simulink model "IARC_Nonlinear_Sensors"  (R2018a)
settings: Solver=ode1  StartTime=0.0  StopTime=20  FixedStep=T  RelTol=1e-3  EnableMultiTasking=on
undefined symbols (not defined in the file): A_1df, A_2df, alpha3, alpha_rp, alpha_x, alpha_z, an1, an1_v, an2, an3, bn1, bn1_v, bn2, bn3, dc_M_x, delta3, Epsilon3, F, g, Gamma1, Gamma2, Gamma3, Gamma4, gamma4_0, gamma_d_x, gamma_rp_0, gamma_x_0, gamma_z_0, Gammax, I, I_add, I_add_time, Jx, Jy, Jyaw, K, k1, k10, k11, k12, k2, k3, k4, k5, k6, k7, k8, k9, Ky, L, Light, LIMIT_CMD_PITCH, LIMIT_CMD_ROLL, LIMIT_CMD_xy, LIMIT_uCMD_HEIGHT, m, m_add, m_add_time, magnitude, MIL ... (+67)
libraries: simulink x131, simulink_extras x5, UAV_Control x4, aerolibwind2 x1
(part 1 of 6)
settings Model: Creator=ahmad  LastModifiedBy=Ahmad
settings SolverCC: AutoInsertRateTranBlk=on
settings DataIOCC: LimitDataPoints=on  SaveFormat=Array
settings OptimizationCC: LifeSpan=inf
settings DebuggingCC: UnderspecifiedInitializationDetection=Classic  MergeDetectMultiDrivingBlocksExec=none  SolverPrmCheckMsg=warning  StateNameClashWarn=warning  SFUnexpectedBacktrackingDiag=warning  SFNoUnconditionalDefaultTransitionDiag=warning  SFExecutionAtInitializationDiag=none
settings HardwareCC: ProdBitPerPointer=32  ProdBitPerSizeT=32  ProdBitPerPtrDiffT=32  ProdLargestAtomicFloat=None  ProdIntDivRoundTo=Undefined  ProdEndianess=Unspecified  ProdWordSize=32  ProdHWDeviceType=32-bit Generic
settings ModelReferenceCC: PropagateSignalLabelsOutOfModel=off
settings CodeAppCC: StateflowObjectComments=on
settings GRTTargetCC: TargetLangStandard=C89/C90 (ANSI)  GeneratePreprocessorConditionals=Disable all
settings ConfigComp: CovMetricSettings=dw  CovHtmlReporting=on  CovSaveCumulativeToWorkspaceVar=on  CovSaveSingleToWorkspaceVar=on  CovExternalEMLEnable=off

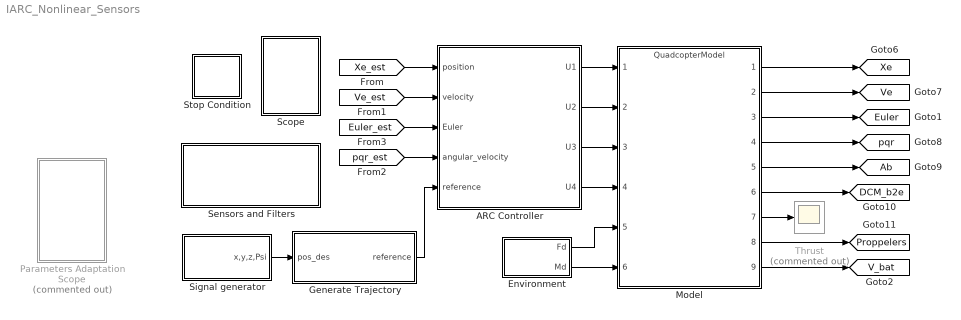
== system IARC_Nonlinear_Sensors ==
  ARC Controller : Subsystem
  Environment : Subsystem
  Generate Trajectory : Subsystem
  Model : ModelReference  ModelNameDialog=QuadcopterModel.slx  SimulationMode=Normal  ModelReferenceVersion=1.100
  Parameters Adaptation Scope : Subsystem  Commented=on
  Scope : Subsystem
  Sensors and Filters : Subsystem
  Signal generator : Subsystem
  Stop Condition : Subsystem
  Thrust : Scope  Commented=on
  tag scope: Ab=global, DCM_b2e=global, Euler=global, Proppelers=global, V_bat=global, Ve=global, Xe=global, pqr=global
  wires:
  Model/3 -> [Euler]
  ARC Controller/1(U1) -> Model/1
  ARC Controller/2(U2) -> Model/2
  ARC Controller/3(U3) -> Model/3
  ARC Controller/4(U4) -> Model/4
  Model/7 -> Thrust/1
  Generate Trajectory/1("reference ") -> ARC Controller/5("reference ")
  Model/4 -> [pqr]
  Model/6 -> [DCM_b2e]
  [Xe_est] -> ARC Controller/1(position)
  [Ve_est] -> ARC Controller/2(velocity)
  [Euler_est] -> ARC Controller/3(Euler)
  [pqr_est] -> ARC Controller/4(angular_velocity)
  Model/1 -> [Xe]
  Model/2 -> [Ve]
  Model/5 -> [Ab]
  Model/8 -> [Proppelers]
  Signal generator/1(x,y,z,Psi) -> Generate Trajectory/1(pos_des)
  Model/9 -> [V_bat]
  Environment/1(Fd) -> Model/5
  Environment/2(Md) -> Model/6

== system IARC_Nonlinear_Sensors/ARC Controller ==
  position : Inport
  velocity : Inport  Port=2
  Euler : Inport  Port=3
  angular_velocity : Inport  Port=4
  "reference " : Inport  Port=5
  Assign : Subsystem
  Attitutde Control : Subsystem
  Forces to decoupled PWM signals : Subsystem  AncestorBlock=UAV_Control/Forces to decoupled PWM signals  mask(Forces2PWMSignals){K=K, Ky=Ky, L=L}
      mask prompts: K "Proppeler Force Coefficient:"; Ky "Proppeler Torque Coefficient:"; L "Arm Length:"
      mask help: Convertes the Quadcopter desired forces and moments to equivalent PWM signal.
      mask Help:
      | Convertes the Quadcopter desired forces and moments to equivalent PWM signal for a specific motors configuration.
      | 
      | Motors indices and rotation direction:
      | 1: back (CW)
      | 2: front (CW)
      | 3: left (CCW)
      | 4: righ (CCW)
      | 
      | parameters:
      | K: Proppeler Force Coefficient (N/(rad/s)^2)
      | Ky: Proppeler Torque Coefficient (N.m/(rad/s)^2)
      | L: Arm Length (m)
      | 
      | Inputs:
      | Fn=F/(4K)
      | Txn=Tx/(2LK)
      | Tyn=Ty/(2LK)
      | Tzn=Tz/(4Ky)
      | 
      | Outputs:
      | u1 =sqrt( Fn + Tyn + Tzn)
      | u2 = sqrt(Fn - Tyn + Tzn)
      | u3 = sqrt(Fn + Txn - Tzn)
      | u4 = sqrt(Fn - Txn - Tzn)
      | 
      | The PWM Duty cylce (ui) is limeted between 0 and 1.
      mask Display:
      | port_label('input',1,'F_{z,des}','texmode','on')
      | port_label('input',2,'\tau_{x,des}','texmode','on')
      | port_label('input',3,'\tau_{y,des}','texmode','on')
      | port_label('input',4,'\tau_{z,des}','texmode','on')
      | port_label('output',1,'U_1','texmode','on')
      | port_label('output',2,'U_2','texmode','on')
      | port_label('output',3,'U_3','texmode','on')
      | port_label('output',4,'U_4','texmode','on')
  Gain1 : Gain
  Gain2 : Gain
  Gain3 : Gain
  LoT : Subsystem
  Mux : Mux
  Position Control : Subsystem
  Saturation1 : Saturate  UpperLimit=LIMIT_CMD_ROLL  LowerLimit=-LIMIT_CMD_ROLL
  Saturation2 : Saturate  UpperLimit=LIMIT_CMD_PITCH  LowerLimit=-LIMIT_CMD_PITCH
  "Thrust Initialization " : Subsystem  AncestorBlock=UAV_Control/Motors Initialization  mask(MotorsInitialization){t0=t0, t1=t1, Sat=Sat, Parameter4=Rate}
      mask prompts: t0 "Initialization delay:"; t1 "Input pass time:"; Sat "Signal saturation during initialization:"; Parameter4 "Signal rate during initialization:"
      mask help: Delays the pass out of the input while passing a warmup rizing signal.
      mask Display:
      | port_label('input',1,'u','texmode','on')
      | port_label('output',1,'y','texmode','on')
  To File4 : ToFile  Commented=on  Filename=U.mat  MatrixName=U  SaveFormat=Timeseries
  To Workspace : ToWorkspace  Commented=on  VariableName=U  SaveFormat=Timeseries  SampleTime=-1
  "U  " : Scope
  take-off flag : Subsystem
  "u1 " : Scope
  U1 : Outport
  U2 : Outport  Port=2
  U3 : Outport  Port=3
  U4 : Outport  Port=4
  tag scope: Fz_des=global, phi_d=global, theta_d=global
  wires:
  Forces to decoupled PWM signals/1(u1) -> Mux/1, U1/1
  Forces to decoupled PWM signals/2(u2) -> Mux/2, U2/1
  Forces to decoupled PWM signals/3(u3) -> Mux/3, U3/1
  Forces to decoupled PWM signals/4(u4) -> Mux/4, U4/1
  take-off flag/2(y2) -> Gain1/1
  Gain2/1 -> Forces to decoupled PWM signals/4(Tz_des)
  "Thrust Initialization "/1(y) -> LoT/1(u)
  take-off flag/3(y3) -> Gain2/1
  [z] -> take-off flag/4(h)
  Mux/1 -> To File4/1, To Workspace/1, "U  "/1
  take-off flag/1("y1 ") -> Gain3/1
  Position Control/2(phi_d) -> Saturation2/1
  Position Control/3(theta_d) -> Saturation1/1
  Saturation2/1 -> [phi_d], Attitutde Control/1(phi_d)
  Saturation1/1 -> [theta_d], Attitutde Control/2(theta_d)
  Attitutde Control/1(Tx) -> take-off flag/1("u1 ")
  Attitutde Control/2(Ty) -> take-off flag/2("u2 ")
  Attitutde Control/3(Tz) -> take-off flag/3(u3)
  Position Control/1(u_1) -> "Thrust Initialization "/1(u)
  LoT/1(y) -> "u1 "/1, [Fz_des], Forces to decoupled PWM signals/1(Fz_des)
  [psi_des] -> Attitutde Control/3(psi_d)
  Gain1/1 -> Forces to decoupled PWM signals/3(Ty_des)
  Gain3/1 -> Forces to decoupled PWM signals/2(Tx_des)
  position/1 -> Assign/1(position)
  velocity/1 -> Assign/2(velocity)
  Euler/1 -> Assign/3(Euler)
  angular_velocity/1 -> Assign/4(angular_velocity)
  "reference "/1 -> Assign/5("reference ")

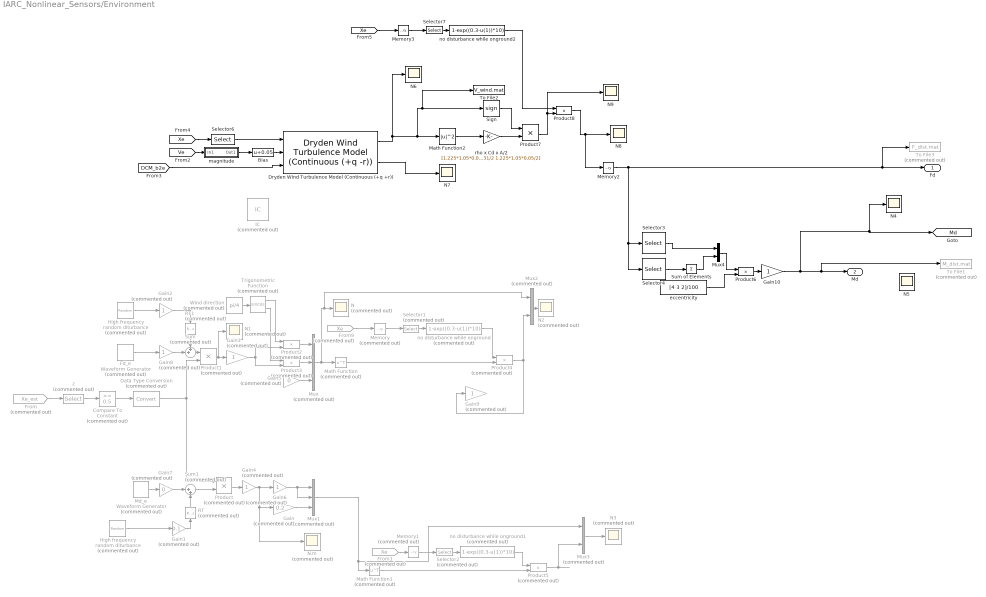
== system IARC_Nonlinear_Sensors/Environment ==
  Bias : Bias  Bias=0.05
  Compare To Constant : simulink/Logic and Bit Operations/Compare To Constant  Commented=on  relop=>=  const=0.5  OutDataTypeStr=boolean
  Data Type Conversion : DataTypeConversion  Commented=on
  Dryden Wind Turbulence Model (Continuous (+q +r)) : aerolibwind2/Dryden Wind Turbulence Model  (Continuous (+q -r))  units=Metric (MKS)  spec=MIL-F-8785C  model=Continuous Dryden (+q +r)  W20=25  Wdeg=30  TurbProb=10^-2 - Light  L_high=533.4  Wingspan=1.5  ts=0.1  Seed=[23341 23342 23443 13344]  T_on=on
      settings: SourceProductName=Aerospace Blockset
  Fd_e : simulink/Sources/Waveform Generator  Commented=on  OutMin=[]  OutMax=[]  OutDataTypeStr=double  SelectedSignal=1  Signals=-sin(0.5,pi/15,pi/3)  BlockNames=MultiportSwitch_6c45d7af92bb48a  SampleTime=T
      settings: SourceProductName=Simulink
  From : From  Commented=on  GotoTag=Xe_est  TagVisibility=global
  From1 : From  Commented=on  GotoTag=Xe  TagVisibility=global
  From9 : From  Commented=on  GotoTag=Xe  TagVisibility=global
  Gain : Gain  Commented=on  Gain=0.2
  Gain1 : Gain  Commented=on  Gain=0.1
  Gain10 : Gain
  Gain{2..4,6,8..9} (6 alike) : Gain  Commented=on
  Gain5 : Gain  Commented=on  Gain=0
  Gain7 : Gain  Commented=on  Gain=0
  High frequency random diturbance : RandomNumber  Commented=on  Variance=0.005  SampleTime=150*T
  "High frequency random diturbance " : RandomNumber  Commented=on  Variance=0.002  SampleTime=150*T
  IC : InitialCondition  Commented=on  Value=[1 0 0; 0 1 0; 0 0 1]
  Math Function : Math  Commented=on  Operator=transpose  SaturateOnIntegerOverflow=on
  Math Function1 : Math  Commented=on  Operator=transpose  SaturateOnIntegerOverflow=on
  Math Function2 : Math  Operator=magnitude^2  SaturateOnIntegerOverflow=on
  Md_e : simulink/Sources/Waveform Generator  Commented=on  OutMin=[]  OutMax=[]  OutDataTypeStr=double  SelectedSignal=1  Signals=sin(0.05,pi/10,0)+sin(0.0005,pi/4,0)#sin(0.001,10*pi,0)  BlockNames=MultiportSwitch_4e1e2af6a5c04c9#MultiportSwitch_b57f3ec1cbf3493  SampleTime=T
      settings: SourceProductName=Simulink
  Memory : Memory  Commented=on
  Memory1 : Memory  Commented=on
  Memory2 : Memory
  Memory3 : Memory
  Mux : Mux  Commented=on  Inputs=3
  Mux1 : Mux  Commented=on  Inputs=3
  Mux2 : Mux  Commented=on  Inputs=2
  Mux3 : Mux  Commented=on  Inputs=2
  Mux4 : Mux  Inputs=2
  N{,1..3} (4 alike) : Scope  Commented=on
  N.m : Scope  Commented=on
  N{4..9} (6 alike) : Scope
  Product{,1..5} (6 alike) : Product  Commented=on
  Product6 : Product
  Product7 : Product
  Product8 : Product
  RT : RateTransition  Commented=on  OutPortSampleTime=0.002
  RT1 : RateTransition  Commented=on  OutPortSampleTime=0.002
  Selector1 : Selector  Commented=on  InputPortWidth=3  IndexOptions=Index vector (dialog)  Indices=3  OutputSizes=1
  Selector2 : Selector  Commented=on  InputPortWidth=3  IndexOptions=Index vector (dialog)  Indices=3  OutputSizes=1
  Selector3 : Selector  InputPortWidth=3  IndexOptions=Index vector (dialog)  Indices=[2 1]  OutputSizes=1
  Selector4 : Selector  InputPortWidth=3  IndexOptions=Index vector (dialog)  Indices=[2 1]  OutputSizes=1
  Selector6 : Selector  InputPortWidth=3  IndexOptions=Index vector (dialog)  Indices=3  OutputSizes=1
  Selector7 : Selector  InputPortWidth=3  IndexOptions=Index vector (dialog)  Indices=3  OutputSizes=1
  Sign : Signum
  Sum : Sum  Commented=on  Inputs=++|
  Sum of Elements : Sum  Inputs=+
  Sum1 : Sum  Commented=on  Inputs=|++
  To File1 : ToFile  Commented=on  Filename=M_dist.mat  MatrixName=M_dist  SaveFormat=Timeseries
  To File2 : ToFile  Filename=V_wind.mat  MatrixName=V_wind  SaveFormat=Timeseries
  To File3 : ToFile  Commented=on  Filename=F_dist.mat  MatrixName=F_dist  SaveFormat=Timeseries
  Trigonometric Function : Trigonometry  Commented=on  Operator=sincos
  Wind direction : Constant  Commented=on  Value=pi/4
  eccentricity : Constant  Value=[4 3 2]/100
  magnitude : Subsystem
  no disturbance while onground : Fcn  Commented=on  Expr=1-exp((0.3-u(1))*10)
  no disturbance while onground1 : Fcn  Commented=on  Expr=1-exp((0.3-u(1))*10)
  no disturbance while onground2 : Fcn  Expr=1-exp((0.3-u(1))*10)
  rho x Cd x A/2 : Gain  Gain=[1.225*1.05*0.0331/2 1.225*1.05*0.0331/2 1.225*1.05*0.05/2]
  z : Selector  Commented=on  InputPortWidth=3  IndexOptions=Index vector (dialog)  Indices=3  OutputSizes=1
  Fd : Outport
  Md : Outport  Port=2
  tag scope: Md=global
  wires:
  From/1 -> z/1
  Compare To Constant/1 -> Data Type Conversion/1
  z/1 -> Compare To Constant/1
  Sum1/1 -> Product/2
  Data Type Conversion/1 -> Product1/2, Product/1
  Fd_e/1 -> Gain8/1
  Mux/1 -> Mux2/1, N/1, Math Function/1
  Mux1/1 -> Math Function1/1, Mux3/1
  Product4/1 -> Mux2/2, Gain9/1
  Product/1 -> Gain4/1
  High frequency random diturbance/1 -> Gain2/1
  Sum/1 -> Product1/1
  Md_e/1 -> Gain7/1
  "High frequency random diturbance "/1 -> Gain1/1
  RT/1 -> Sum1/2
  RT1/1 -> Sum/1
  Gain/1 -> Mux1/3
  Gain1/1 -> RT/1
  Gain2/1 -> RT1/1
  Gain4/1 -> Gain6/1, Gain/1, N.m/1
  Gain5/1 -> Mux/3
  Wind direction/1 -> Trigonometric Function/1
  Product2/1 -> Mux/1
  Product3/1 -> Mux/2
  Trigonometric Function/1 -> Product2/1
  Trigonometric Function/2 -> Product3/1
  Gain3/1 -> Product3/2, Product2/2
  Product1/1 -> N1/1, Gain3/1
  Gain6/1 -> Mux1/2, Mux1/1
  Math Function/1 -> Product4/2
  From9/1 -> Memory/1
  Selector1/1 -> no disturbance while onground/1
  no disturbance while onground/1 -> Product4/1
  no disturbance while onground1/1 -> Product5/1
  Selector2/1 -> no disturbance while onground1/1
  From1/1 -> Memory1/1
  Math Function1/1 -> Product5/2
  Memory/1 -> Selector1/1
  Memory1/1 -> Selector2/1
  Product5/1 -> Mux3/2
  Mux2/1 -> N2/1
  Mux3/1 -> N3/1
  Gain7/1 -> Sum1/1
  Gain8/1 -> Sum/2
  Product6/1 -> Gain10/1
  eccentricity/1 -> Product6/2
  Selector3/1 -> Mux4/1
  Selector4/1 -> Sum of Elements/1
  Mux4/1 -> Product6/1
  Sum of Elements/1 -> Mux4/2
  Gain10/1 -> N4/1, [Md], To File1/1, Md/1
  magnitude/1(Out1) -> Bias/1
  Dryden Wind Turbulence Model (Continuous (+q +r))/2 -> N7/1
  [Xe] -> Selector6/1
  [Ve] -> magnitude/1(In1)
  Selector6/1 -> Dryden Wind Turbulence Model (Continuous (+q +r))/1
  Dryden Wind Turbulence Model (Continuous (+q +r))/1 -> N6/1, To File2/1, Sign/1, Math Function2/1
  [DCM_b2e] -> Dryden Wind Turbulence Model (Continuous (+q +r))/3
  Bias/1 -> Dryden Wind Turbulence Model (Continuous (+q +r))/2
  Math Function2/1 -> rho x Cd x A/2/1
  rho x Cd x A/2/1 -> Product7/2
  Sign/1 -> Product7/1
  Memory3/1 -> Selector7/1
  no disturbance while onground2/1 -> Product8/1
  Selector7/1 -> no disturbance while onground2/1
  [Xe] -> Memory3/1
  Product8/1 -> N8/1, Memory2/1
  Product7/1 -> N9/1, Product8/2
  Memory2/1 -> To File3/1, Fd/1, Selector4/1, Selector3/1

== system IARC_Nonlinear_Sensors/Generate Trajectory ==
  pos_des : Inport
  Bias : Bias  Commented=on  Bias=-15
  Bias1 : Bias  Bias=Zg
  Clock2 : Clock  Commented=on
  Compare To Constant1 : simulink/Logic and Bit Operations/Compare To Constant  Commented=on  relop=>=  const=15  OutDataTypeStr=boolean
  Compare To Constant2 : simulink/Logic and Bit Operations/Compare To Constant  Commented=on  relop=<=  const=20  OutDataTypeStr=boolean
  Demux : Demux
  Logical Operator : Logic  Commented=on  AllPortsSameDT=off  OutDataTypeStr=boolean
  Mux : Mux
  Product1 : Product  Commented=on
  Rate Limiter1 : RateLimiter
  Rate Limiter2 : RateLimiter
  Rate Limiter3 : RateLimiter  RisingSlewLimit=2  FallingSlewLimit=-2
  Sine Wave2 : Sin  Commented=on  TimeSource=Use external signal  Frequency=2*pi  SampleTime=0
  Sum4 : Sum  Inputs=++|
  Transfer Fcn11 : TransferFcn  Denominator=conv(conv(conv([0.2 1],[0.2 1]),[0.2 1]),[0.2 1])
  Transfer Fcn14 : TransferFcn  Denominator=conv(conv(conv([0.2 1],[0.2 1]),[0.2 1]),[0.2 1])
  Transfer Fcn17 : TransferFcn  Denominator=conv([0.2 1],[0.2 1])
  Transfer Fcn6 : TransferFcn  Denominator=conv(conv(conv([0.2 1],[0.2 1]),[0.2 1]),[0.2 1])
  Transfer Fcn8 : TransferFcn  Commented=on  Denominator=conv(conv(conv(conv(conv(conv(conv([0.2 1],[0.2 1]),[0.2 1]),[0.2 1]),[0.2 1]),[0.2 1]),[0.2 1]),[0.2 1])
  adjust_for_heading3 : Subsystem  Commented=on
  des psi : Scope  Commented=on
  des x : Scope  Commented=on
  des x3 : Scope  Commented=on
  des y : Scope  Commented=on
  des z : Scope  Commented=on
  steady takeoff (x) : Subsystem  Commented=on
  steady takeoff (y) : Subsystem  Commented=on
  "reference " : Outport
  wires:
  Bias1/1 -> des z/1, Mux/3  "z_des"
  Demux/2 -> Rate Limiter1/1  "y_des"
  pos_des/1 -> Demux/1
  Sum4/1 -> Mux/1, des x/1
  Product1/1 -> Transfer Fcn8/1
  Clock2/1 -> Compare To Constant2/1, Bias/1, Compare To Constant1/1
  Logical Operator/1 -> Product1/2
  Sine Wave2/1 -> Product1/1
  Transfer Fcn8/1 -> ?
  Bias/1 -> Sine Wave2/1
  Compare To Constant2/1 -> Logical Operator/1
  Compare To Constant1/1 -> Logical Operator/2
  Demux/4 -> Transfer Fcn17/1  "psi_des"
  Demux/1 -> Rate Limiter2/1, des x3/1  "x_des"
  Mux/1 -> "reference "/1
  Demux/3 -> Rate Limiter3/1  "z_des"
  Transfer Fcn11/1 -> Bias1/1  "z_des"
  Rate Limiter3/1 -> Transfer Fcn11/1
  Rate Limiter2/1 -> Transfer Fcn6/1  "x_des"
  Transfer Fcn6/1 -> Sum4/2
  Transfer Fcn14/1 -> Mux/2, des y/1
  Rate Limiter1/1 -> Transfer Fcn14/1  "y_des"
  Transfer Fcn17/1 -> Mux/4, des psi/1

== system IARC_Nonlinear_Sensors/Parameters Adaptation Scope ==
  Mux{,1..4} (5 alike) : Mux
  Subsystem : Subsystem
  Subsystem1 : Subsystem
  Subsystem2 : Subsystem
  m : Scope
  max : Constant  Value=theta1_Max
  max1 : Constant  Value=theta2_Max
  max2 : Constant  Value=theta3_Max(1)
  max3 : Constant  Value=theta4_Max
  max4 : Constant  Value=theta3_Max(2)
  min : Constant  Value=theta1_Min
  min1 : Constant  Value=theta2_Min
  min2 : Constant  Value=theta3_Min(1)
  min3 : Constant  Value=theta4_Min
  min4 : Constant  Value=theta3_Min(2)
  real : Constant  Value=theta1
  real1 : Constant  Value=theta2
  real2 : Constant  Value=theta3(1)
  real3 : Constant  Value=theta4
  real4 : Constant  Value=theta3(2)
  theta1 1/Iy : Scope
  theta2 1/Ix : Scope
  theta3_1 1/m : Scope
  theta3_2 d0 : Scope
  theta4 1/Iz : Scope
  wires:
  min1/1 -> Mux1/4
  max1/1 -> Mux1/1
  real2/1 -> Mux2/2
  Mux1/1 -> theta2 1/Ix/1
  Mux2/1 -> Subsystem2/1(" "), Subsystem/1(" ")
  max2/1 -> Mux2/1
  min2/1 -> Mux2/4
  [theta2_est] -> Mux1/3
  real1/1 -> Mux1/2
  Mux/1 -> theta1 1/Iy/1
  real/1 -> Mux/2
  [theta4_est] -> Mux3/3
  [theta1_est] -> Mux/3
  min/1 -> Mux/4
  Mux3/1 -> theta4 1/Iz/1
  max3/1 -> Mux3/1
  real3/1 -> Mux3/2
  min3/1 -> Mux3/4
  max/1 -> Mux/1
  real4/1 -> Mux4/2
  Mux4/1 -> Subsystem1/1(" ")
  max4/1 -> Mux4/1
  min4/1 -> Mux4/4
  [theta3_est] -> Mux2/3
  [theta3_est] -> Mux4/3
  Subsystem/1("  ") -> m/1
  Subsystem1/1("  ") -> theta3_2 d0/1
  Subsystem2/1("  ") -> theta3_1 1/m/1

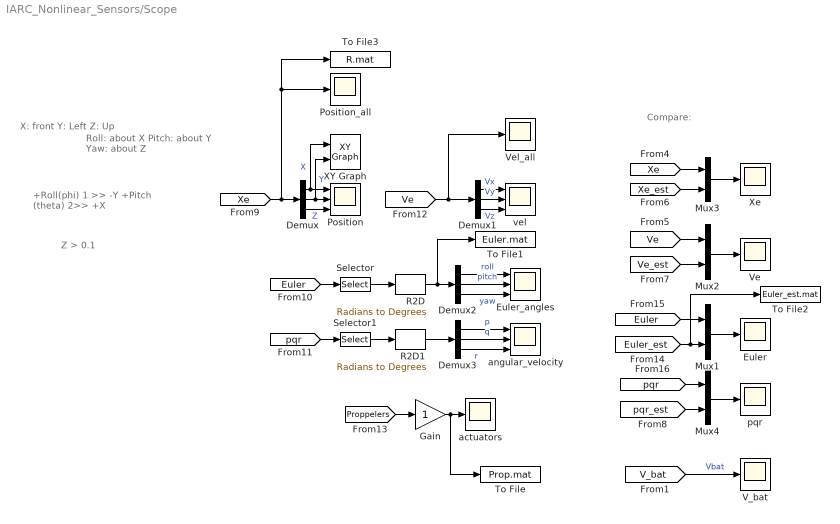
== system IARC_Nonlinear_Sensors/Scope ==
  note: Compare:
  note: +Roll(phi) 1 >> -Y
      | +Pitch (theta) 2>> +X
  note: Roll: about X
      | Pitch: about Y
      | Yaw: about Z
  note: Z > 0.1
  note: X: front
      | Y: Left
      | Z: Up
  Demux{,1..3} (4 alike) : Demux  Outputs=3
  "Euler " : Scope
  Euler_angles : Scope  NumInputPorts=3
  Gain : Gain
  Mux{1..4} (4 alike) : Mux  Inputs=2
  Position : Scope  NumInputPorts=3
  Position_all : Scope
  R2D : simulink_extras/Transformations/Radians to Degrees
  R2D1 : simulink_extras/Transformations/Radians to Degrees
  Selector : Selector  InputPortWidth=3  IndexOptions=Index vector (dialog)  Indices=[1 2 3]  OutputSizes=1
  Selector1 : Selector  InputPortWidth=3  IndexOptions=Index vector (dialog)  Indices=[1 2 3]  OutputSizes=1
  To File : ToFile  Filename=Prop.mat  MatrixName=Prop  SaveFormat=Timeseries
  To File1 : ToFile  Filename=Euler.mat  MatrixName=Euler  SaveFormat=Timeseries
  To File2 : ToFile  Filename=Euler_est.mat  MatrixName=Euler_est  SaveFormat=Timeseries
  To File3 : ToFile  Filename=R.mat  MatrixName=R  SaveFormat=Timeseries
  V_bat : Scope
  Ve : Scope
  Vel_all : Scope
  XY Graph : simulink/Sinks/XY Graph  xmin=-3  xmax=3  ymin=-3  ymax=3  st=1/100
  Xe : Scope
  actuators : Scope
  angular_velocity : Scope  NumInputPorts=3
  "pqr " : Scope
  vel : Scope  NumInputPorts=3
  wires:
  [pqr_est] -> Mux4/2
  Mux1/1 -> "Euler "/1
  [Euler] -> Selector/1
  [Ve] -> Vel_all/1, Demux1/1
  Demux2/3 -> Euler_angles/3  "yaw"
  [Xe_est] -> Mux3/2
  [Euler] -> Mux1/1
  [pqr] -> Selector1/1
  Mux4/1 -> "pqr "/1
  Selector1/1 -> R2D1/1
  [Ve] -> Mux2/1
  [Xe] -> To File3/1, Position_all/1, Demux/1
  [Proppelers] -> Gain/1
  Mux2/1 -> Ve/1
  Demux2/1 -> Euler_angles/1  "roll"
  Mux3/1 -> Xe/1
  Demux3/3 -> angular_velocity/3  "r"
  R2D1/1 -> Demux3/1
  Selector/1 -> R2D/1
  Demux1/1 -> vel/1  "Vx"
  Demux1/2 -> vel/2  "Vy"
  [Ve_est] -> Mux2/2
  Demux3/2 -> angular_velocity/2  "q"
  Gain/1 -> To File/1, actuators/1
  [pqr] -> Mux4/1
  Demux/3 -> Position/3  "Z"
  Demux/1 -> Position/1, XY Graph/1  "X"
  Demux1/3 -> vel/3  "Vz"
  R2D/1 -> To File1/1, Demux2/1
  [Xe] -> Mux3/1
  Demux3/1 -> angular_velocity/1  "p"
  Demux/2 -> XY Graph/2, Position/2  "Y"
  Demux2/2 -> Euler_angles/2  "pitch"
  [Euler_est] -> To File2/1, Mux1/2
  [V_bat] -> V_bat/1  "Vbat"

== system IARC_Nonlinear_Sensors/Sensors and Filters ==
  Data processing : Subsystem
  Rotation Angles to Angular transformation matrix earth to body Rotation Order: ZXY : UAV_Control/Rotation Angles to Angular transformation matrix earth to body Rotation Order: ZXY
      settings: SourceProductName=UAV_Control
  Sensors : Subsystem
  tag scope: Euler_est=global, Rr_est=global, Ve_est=global, Xe_est=global, pqr_est=global, pqr_gyro=global
  wires:
  Data processing/4("p,q,r_est ") -> [pqr_est]
  [Euler] -> Sensors/4(Euler)
  Sensors/3("p,q,r ") -> Data processing/3(p,q,r)
  [pqr] -> Sensors/1(p,q,r)
  [Xe] -> Sensors/3(Xe)
  [DCM_b2e] -> Sensors/5(DCM_b2e)
  Sensors/1(Acc) -> Data processing/1(Acc)
  Sensors/2(OptiTrack) -> Data processing/2(OptiTrack)
  Data processing/2(Ve_est) -> [Ve_est]
  Data processing/1(Xe_est) -> [Xe_est]
  [Ab] -> Sensors/2(Ab)
  Data processing/3(p,q,r_gyro) -> [pqr_gyro]
  Rotation Angles to Angular transformation matrix earth to body Rotation Order: ZXY/1 -> [Rr_est]
  Data processing/5(" Euler_est") -> Rotation Angles to Angular transformation matrix earth to body Rotation Order: ZXY/1, [Euler_est]

== system IARC_Nonlinear_Sensors/Signal generator ==
  Mux1 : Mux
  Position2 : Scope  Commented=on
  Rate Transition : RateTransition  Commented=on
  Repeating Sequence Stair : simulink/Sources/Repeating Sequence Stair  Commented=on  OutValues=[0 0 1 0 0 -1 0 1].'  tsamp=T*500*5  OutMin=[]  OutMax=[]  OutDataTypeStr=double  OutputDataTypeScalingMode=double  OutDataType=fixdt(0,8)  ConRadixGroup=Best Precision: Vector-wise  OutScaling=2^-12
  X Des : Scope  Commented=on
  X_des : Subsystem
  Y Des : Scope  Commented=on
  Y_des : Subsystem
  Yaw_des : Subsystem
  Z_des : Subsystem
  x,y,z,Psi : Outport
  wires:
  Rate Transition/1 -> Position2/1
  Repeating Sequence Stair/1 -> Rate Transition/1  "y_des"
  Mux1/1 -> x,y,z,Psi/1
  Z_des/1(z_des) -> Mux1/3
  X_des/1(x_des) -> X Des/1, Mux1/1
  Y_des/1(x_des) -> Y Des/1, Mux1/2
  Yaw_des/1(Out1) -> Mux1/4

== system IARC_Nonlinear_Sensors/Stop Condition ==
  Abs : Abs
  Abs1 : Abs
  Assertion : Assertion  AssertionFailFcn=msgbox('Low Voltage!')
  Assertion1 : Assertion  AssertionFailFcn=msgbox('Crash!')
  Compare To Constant : simulink/Logic and Bit Operations/Compare To Constant  relop=>=  const=3.0  OutDataTypeStr=boolean
  Compare To Constant1 : simulink/Logic and Bit Operations/Compare To Constant  relop=>=  const=3.0  OutDataTypeStr=boolean
  Compare To Constant2 : simulink/Logic and Bit Operations/Compare To Constant  relop=>=  const=3.0  OutDataTypeStr=boolean
  Compare To Constant3 : simulink/Logic and Bit Operations/Compare To Constant  relop=<=  const=Zg  OutDataTypeStr=boolean
  Compare To Constant4 : simulink/Logic and Bit Operations/Compare To Constant  relop=<  const=-1  OutDataTypeStr=boolean
  Compare To Constant5 : simulink/Logic and Bit Operations/Compare To Constant  relop=>=  const=Zg+10/100  OutDataTypeStr=boolean
  Compare To Constant6 : simulink/Logic and Bit Operations/Compare To Constant  relop=<  const=9  OutDataTypeStr=boolean
  Demux : Demux  Outputs=3
  Logical Operator : Logic  Inputs=3  AllPortsSameDT=off  OutDataTypeStr=boolean
  Logical Operator1 : Logic  Operator=OR  Inputs=4  AllPortsSameDT=off  OutDataTypeStr=boolean
  Logical Operator2 : Logic  Operator=NOT  AllPortsSameDT=off  OutDataTypeStr=boolean
  Logical Operator3 : Logic  Operator=NOT  AllPortsSameDT=off  OutDataTypeStr=boolean
  Vz : Selector  InputPortWidth=3  IndexOptions=Index vector (dialog)  Indices=3  OutputSizes=1
  st : Scope  Commented=on
  wires:
  Demux/1 -> Abs/1
  Compare To Constant/1 -> Logical Operator1/1
  Vz/1 -> Compare To Constant4/1
  Demux/3 -> Compare To Constant3/1, Compare To Constant2/1
  Compare To Constant3/1 -> Logical Operator/1
  Abs/1 -> Compare To Constant/1
  [Xe] -> Demux/1
  Compare To Constant1/1 -> Logical Operator1/2
  Abs1/1 -> Compare To Constant1/1
  Logical Operator1/1 -> Logical Operator2/1
  Demux/2 -> Abs1/1
  Logical Operator/1 -> st/1, Logical Operator1/4
  Compare To Constant2/1 -> Logical Operator1/3
  Compare To Constant4/1 -> Logical Operator/2
  [Ve] -> Vz/1
  [z_des] -> Compare To Constant5/1
  Compare To Constant5/1 -> Logical Operator/3
  [V_bat] -> Compare To Constant6/1
  Compare To Constant6/1 -> Logical Operator3/1
  Logical Operator2/1 -> Assertion1/1
  Logical Operator3/1 -> Assertion/1

== system IARC_Nonlinear_Sensors/ARC Controller/Assign ==
  position : Inport
  velocity : Inport  Port=2
  Euler : Inport  Port=3
  angular_velocity : Inport  Port=4
  "reference " : Inport  Port=5
  Demux{,1,3..4} (4 alike) : Demux  Outputs=3
  Demux2 : Demux
  tag scope: phi=global, phi_dot=global, psi=global, psi_des=global, psi_dot=global, theta=global, theta_dot=global, x=global, x_des=global, x_dot=global, y=global, y_des=global, y_dot=global, z=global, z_des=global, z_dot=global
  wires:
  position/1 -> Demux/1
  Demux2/1 -> [x_des]
  Demux1/3 -> [psi]
  Demux1/2 -> [theta]
  Demux/3 -> [z]
  Euler/1 -> Demux1/1
  Demux4/3 -> [z_dot]
  "reference "/1 -> Demux2/1
  Demux2/4 -> [psi_des]
  Demux3/3 -> [psi_dot]
  Demux/2 -> [y]
  velocity/1 -> Demux4/1
  Demux3/1 -> [phi_dot]
  Demux4/2 -> [y_dot]
  Demux1/1 -> [phi]
  Demux4/1 -> [x_dot]
  Demux/1 -> [x]
  Demux2/2 -> [y_des]
  Demux2/3 -> [z_des]
  Demux3/2 -> [theta_dot]
  angular_velocity/1 -> Demux3/1

== system IARC_Nonlinear_Sensors/ARC Controller/Attitutde Control ==
  phi_d : Inport
  theta_d : Inport  Port=2
  psi_d : Inport  Port=3
  Add : Sum  Commented=on  Inputs=--+-++
  Product : Product  Commented=on  Multiplication=Matrix(*)
  Product1 : Product  Commented=on  Multiplication=Matrix(*)
  Product2 : Product  Commented=on  Multiplication=Matrix(*)
  Subsystem : Subsystem  Commented=on
  Yaw control : Subsystem
  pitch control : Subsystem
  roll control : Subsystem
  u_{1..8} (8 alike) : Scope  Commented=on
  Tx : Outport
  Ty : Outport  Port=2
  Tz : Outport  Port=3
  wires:
  theta_d/1 -> pitch control/1(theta_d)
  phi_d/1 -> roll control/1(phi_d)
  Subsystem/1("inv(g) ") -> u_4/1, Product/1
  Subsystem/2("f ") -> u_1/1, Add/1
  Subsystem/3(D) -> u_6/1, Add/2
  Product1/1 -> u_5/1, Add/3
  Subsystem/4(k1) -> Product1/1
  Subsystem/6(e1) -> Product1/2, u_8/1, Add/5
  Product2/1 -> u_7/1, Add/4
  Subsystem/5(k2) -> Product2/1
  Subsystem/7(e2) -> Product2/2
  Add/1 -> Product/2
  Subsystem/8(X_ddot) -> u_3/1, Add/6
  Product/1 -> u_2/1
  roll control/1(U4 (N.m)) -> Tx/1
  pitch control/1(U5 (N.m)) -> Ty/1
  psi_d/1 -> Yaw control/1(psi_d)
  Yaw control/1(U6 (N.m)) -> Tz/1

== system IARC_Nonlinear_Sensors/ARC Controller/Forces to decoupled PWM signals ==
  Fz_des : Inport
  Tx_des : Inport  Port=2
  Ty_des : Inport  Port=3
  Tz_des : Inport  Port=4
  Gain : Gain  Commented=on  Gain=1/2
  Gain1 : Gain  Commented=on  Gain=1/4
  Gain2 : Gain  Gain=1/(L*2*K)
  Gain3 : Gain  Gain=1/(4*Ky)
  Gain4 : Gain  Gain=1/(L*2*K)
  Gain5 : Gain  Gain=1/(4*K)
  Gain6 : Gain  Commented=on  Gain=1/2
  Gain7 : Gain  Commented=on  Gain=1/4
  Mux : Mux
  Saturation{1..4} (4 alike) : Saturate  UpperLimit=1  LowerLimit=0
  Sqrt{,1..3} (4 alike) : Sqrt  Operator=signedSqrt  OutputSignalType=real  SaturateOnIntegerOverflow=on
  u1^2 - Back (PWM command) : Fcn  Expr=u(1)+u(3)+u(4)
  u2^2 - Front (PWM command) : Fcn  Expr=u(1)-u(3)+u(4)
  u3^2 - Left (PWM command) : Fcn  Expr=u(1)+u(2)-u(4)
  u4^2 - Right (PWM command) : Fcn  Expr=u(1)-u(2)-u(4)
  u1 : Outport
  u2 : Outport  Port=2
  u3 : Outport  Port=3
  u4 : Outport  Port=4
  wires:
  Tx_des/1 -> Gain2/1
  Fz_des/1 -> Gain5/1
  Ty_des/1 -> Gain4/1
  Tz_des/1 -> Gain3/1
  Mux/1 -> u4^2 - Right (PWM command)/1, u3^2 - Left (PWM command)/1, u2^2 - Front (PWM command)/1, u1^2 - Back (PWM command)/1
  Gain2/1 -> Mux/2
  Gain4/1 -> Mux/3
  Gain3/1 -> Mux/4
  Gain5/1 -> Mux/1
  Saturation4/1 -> u1/1
  Saturation2/1 -> u3/1
  Saturation3/1 -> u2/1
  Saturation1/1 -> u4/1
  u1^2 - Back (PWM command)/1 -> Sqrt/1
  u2^2 - Front (PWM command)/1 -> Sqrt1/1
  u3^2 - Left (PWM command)/1 -> Sqrt2/1
  u4^2 - Right (PWM command)/1 -> Sqrt3/1
  Sqrt/1 -> Saturation4/1
  Sqrt3/1 -> Saturation1/1
  Sqrt2/1 -> Saturation2/1
  Sqrt1/1 -> Saturation3/1

== system IARC_Nonlinear_Sensors/ARC Controller/LoT ==
  u : Inport
  Gain : Gain  Gain=0
  Product : Product
  Step : Step  Time=40  SampleTime=0
  Sum : Sum  Inputs=-+|
  y : Outport
  wires:
  Step/1 -> Product/1
  Product/1 -> Sum/1
  u/1 -> Gain/1, Sum/2
  Sum/1 -> y/1
  Gain/1 -> Product/2

== system IARC_Nonlinear_Sensors/ARC Controller/Position Control ==
  Coupling : Subsystem
  X control : Subsystem
  Y control : Subsystem
  Z control : Subsystem
  phi_des : Scope
  theta_des : Scope
  u1 : Scope
  u_1 : Outport
  phi_d : Outport  Port=2
  theta_d : Outport  Port=3
  wires:
  [psi_des] -> Coupling/4(psi_d)
  X control/1(U1 (m/s^2)) -> Coupling/1(U1)
  Y control/1(U2 (m/s^2)) -> Coupling/2(U2)
  Z control/1(U3 (m/s^2)) -> Coupling/3(U3)
  Coupling/2(phi_d (rad)) -> phi_d/1, phi_des/1
  Coupling/3(theta_d (rad)) -> theta_des/1, theta_d/1
  Coupling/1(u1 (N)) -> u_1/1, u1/1

== system IARC_Nonlinear_Sensors/ARC Controller/Thrust Initialization  ==
  u : Inport
  Clock : Clock
  Compare To Constant1 : simulink/Logic and Bit Operations/Compare To Constant  relop=<=  const=t1  OutDataTypeStr=boolean
  Compare To Constant2 : simulink/Logic and Bit Operations/Compare To Constant  relop=>=  const=t0  OutDataTypeStr=boolean
  Constant : Constant  Value=0
  Gain : Gain  Gain=Rate
  Saturation : Saturate  UpperLimit=Sat  LowerLimit=0
  Scope : Scope
  Scope1 : Scope
  Switch : Switch  Criteria=u2 > Threshold  Threshold=0.5
  Switch1 : Switch  Criteria=u2 > Threshold  Threshold=0.5
  y : Outport
  wires:
  Switch/1 -> Scope/1, Switch1/1
  Switch1/1 -> y/1, Scope1/1
  Compare To Constant1/1 -> Switch1/2
  Constant/1 -> Switch/3
  Saturation/1 -> Switch/1
  Gain/1 -> Saturation/1
  Compare To Constant2/1 -> Switch/2
  Clock/1 -> Gain/1, Compare To Constant2/1, Compare To Constant1/1
  u/1 -> Switch1/3

== system IARC_Nonlinear_Sensors/ARC Controller/take-off flag ==
  "u1 " : Inport
  "u2 " : Inport  Port=2
  u3 : Inport  Port=3
  h : Inport  Port=4
  Constant : Constant  Value=[0 0 0]
  Demux : Demux  Outputs=3
  Mux : Mux  Inputs=3
  Switch : Switch  Criteria=u2 > Threshold  Threshold=X0(3)+2/100
  "y1 " : Outport
  y2 : Outport  Port=2
  y3 : Outport  Port=3
  wires:
  Constant/1 -> Switch/3
  Demux/1 -> "y1 "/1
  Mux/1 -> Switch/1
  "u1 "/1 -> Mux/1
  "u2 "/1 -> Mux/2
  u3/1 -> Mux/3
  h/1 -> Switch/2
  Switch/1 -> Demux/1
  Demux/3 -> y3/1
  Demux/2 -> y2/1

== system IARC_Nonlinear_Sensors/Environment/magnitude ==
  In1 : Inport
  Math Function2 : Math  Operator=magnitude^2  SaturateOnIntegerOverflow=on
  Sqrt : Sqrt  SaturateOnIntegerOverflow=on
  Sum of Elements1 : Sum  Inputs=+
  Out1 : Outport
  wires:
  Sum of Elements1/1 -> Sqrt/1
  Math Function2/1 -> Sum of Elements1/1
  Sqrt/1 -> Out1/1
  In1/1 -> Math Function2/1

== system IARC_Nonlinear_Sensors/Generate Trajectory/adjust_for_heading3 ==
  x_w_des : Inport
  y_w_des : Inport  Port=2
  adjust_for_heading1 : Subsystem
  adjust_for_heading3 : Subsystem
  x_des_adj : Outport
  y_des_adj : Outport  Port=2
  wires:
  y_w_des/1 -> adjust_for_heading3/2(y_e_d), adjust_for_heading1/2(y_e_d)
  [psi] -> adjust_for_heading3/3(yaw), adjust_for_heading1/3(yaw)
  x_w_des/1 -> adjust_for_heading3/1(x_e_d), adjust_for_heading1/1(x_e_d)
  adjust_for_heading1/1(adj) -> x_des_adj/1
  adjust_for_heading3/1(adj) -> y_des_adj/1

== system IARC_Nonlinear_Sensors/Generate Trajectory/steady takeoff (x) ==
  u : Inport
  Compare To Constant : simulink/Logic and Bit Operations/Compare To Constant  relop=>=  const=Safe_hight  OutDataTypeStr=boolean
  Data Type Conversion : DataTypeConversion
  Mux : Mux  Inputs=3
  Switch : Switch  Criteria=u2 > Threshold  Threshold=0.5
  Triggered Subsystem1 : Subsystem  TreatAsAtomicUnit=on
  Triggered Subsystem2 : Subsystem  TreatAsAtomicUnit=on
  start from initial position : Sum  Inputs=|++
  z_des{1,4..5,7} (4 alike) : Scope
  y : Outport
  wires:
  Triggered Subsystem2/1("  ") -> z_des7/1, Mux/2, Switch/3, start from initial position/2
  [takeoff] -> Triggered Subsystem2/Trigger
  start from initial position/1 -> Mux/1, Switch/1
  [z] -> Compare To Constant/1
  Switch/1 -> Mux/3, y/1
  [x] -> Triggered Subsystem2/1(" "), z_des5/1
  Triggered Subsystem1/1("  ") -> z_des4/1, Switch/2
  Compare To Constant/1 -> Data Type Conversion/1
  Data Type Conversion/1 -> Triggered Subsystem1/Trigger, Triggered Subsystem1/1(" ")
  Mux/1 -> z_des1/1
  u/1 -> start from initial position/1

== system IARC_Nonlinear_Sensors/Generate Trajectory/steady takeoff (y) ==
  u : Inport
  Compare To Constant : simulink/Logic and Bit Operations/Compare To Constant  relop=>=  const=Safe_hight  OutDataTypeStr=uint8
  Data Type Conversion : DataTypeConversion
  Switch : Switch  Criteria=u2 > Threshold  Threshold=0.5
  Triggered Subsystem1 : Subsystem  TreatAsAtomicUnit=on
  Triggered Subsystem2 : Subsystem  TreatAsAtomicUnit=on
  start from initial position : Sum  Inputs=|++
  z_des4 : Scope
  z_des5 : Scope
  z_des7 : Scope
  y : Outport
  wires:
  Compare To Constant/1 -> Data Type Conversion/1
  Triggered Subsystem1/1("  ") -> Switch/2, z_des4/1
  [y] -> Triggered Subsystem2/1(" "), z_des5/1
  Switch/1 -> y/1
  [z] -> Compare To Constant/1
  start from initial position/1 -> Switch/1
  [takeoff] -> Triggered Subsystem2/Trigger
  Triggered Subsystem2/1("  ") -> start from initial position/2, Switch/3, z_des7/1
  Data Type Conversion/1 -> Triggered Subsystem1/Trigger, Triggered Subsystem1/1(" ")
  u/1 -> start from initial position/1

== system IARC_Nonlinear_Sensors/Parameters Adaptation Scope/Subsystem ==
  " " : Inport
  Demux : Demux  Outputs=5
  Math Function1 : Math  Operator=reciprocal  SaturateOnIntegerOverflow=on
  Mux5 : Mux
  Terminator : Terminator
  "  " : Outport
  wires:
  Demux/2 -> Mux5/2
  " "/1 -> Demux/1
  Demux/5 -> Mux5/4
  Demux/3 -> Mux5/3
  Demux/1 -> Mux5/1
  Demux/4 -> Terminator/1
  Mux5/1 -> Math Function1/1
  Math Function1/1 -> "  "/1

== system IARC_Nonlinear_Sensors/Parameters Adaptation Scope/Subsystem1 ==
  " " : Inport
  Demux : Demux  Outputs=5
  Mux5 : Mux
  Terminator : Terminator
  "  " : Outport
  wires:
  Demux/2 -> Mux5/2
  " "/1 -> Demux/1
  Demux/5 -> Mux5/4
  Demux/3 -> Terminator/1
  Demux/1 -> Mux5/1
  Demux/4 -> Mux5/3
  Mux5/1 -> "  "/1

== system IARC_Nonlinear_Sensors/Parameters Adaptation Scope/Subsystem2 ==
  " " : Inport
  Demux : Demux  Outputs=5
  Mux5 : Mux
  Terminator : Terminator
  "  " : Outport
  wires:
  Mux5/1 -> "  "/1
  Demux/4 -> Terminator/1
  Demux/1 -> Mux5/1
  Demux/3 -> Mux5/3
  Demux/5 -> Mux5/4
  " "/1 -> Demux/1
  Demux/2 -> Mux5/2

== system IARC_Nonlinear_Sensors/Sensors and Filters/Data processing ==
  Acc : Inport
  OptiTrack : Inport  Port=2
  p,q,r : Inport  Port=3
  Estimate Attitude : Subsystem
  Estimate Position : Subsystem
  "Euler " : Selector  InputPortWidth=8  IndexOptions=Index vector (dialog)  Indices=[4 5 6]  OutputSizes=1
  OptiTrack1 : InportShadow  Port=2
  Xe_est : Outport
  Ve_est : Outport  Port=2
  p,q,r_gyro : Outport  Port=3
  "p,q,r_est " : Outport  Port=4
  " Euler_est" : Outport  Port=5
  wires:
  OptiTrack1/1 -> "Euler "/1
  Acc/1 -> Estimate Attitude/1(Acc)
  p,q,r/1 -> Estimate Attitude/2(p,q,r)
  "Euler "/1 -> Estimate Attitude/3(Euler)
  Estimate Attitude/2(p,q,r_f) -> "p,q,r_est "/1
  Estimate Attitude/3(" Euler") -> " Euler_est"/1
  OptiTrack/1 -> Estimate Position/1(OptiTrack)
  Estimate Position/1(Xe) -> Xe_est/1
  Estimate Position/2(Ve) -> Ve_est/1
  Estimate Attitude/1(p,q,r_g) -> p,q,r_gyro/1

== system IARC_Nonlinear_Sensors/Sensors and Filters/Sensors ==
  note: Gyro noise destroys the estimation
  note: Acc noise does not affect estimation
  p,q,r : Inport
  Ab : Inport  Port=2
  Xe : Inport  Port=3
  Euler : Inport  Port=4
  DCM_b2e : Inport  Port=5
  Accelerometer : Subsystem
  Gyro : Subsystem
  "OptiTrack " : Subsystem
  acc : Scope  Commented=on
  optiTrack : Scope  Commented=on
  pqr : Scope  Commented=on
  Acc : Outport
  OptiTrack : Outport  Port=2
  "p,q,r " : Outport  Port=3
  wires:
  Xe/1 -> "OptiTrack "/1(Xe)
  Ab/1 -> Accelerometer/1(Ab)
  p,q,r/1 -> Gyro/1(p,q,r)
  Euler/1 -> "OptiTrack "/2(Euler)
  DCM_b2e/1 -> Accelerometer/2(DCM_b2e)
  Accelerometer/1(Acc) -> acc/1, Acc/1
  Gyro/1("p,q,r ") -> pqr/1, "p,q,r "/1
  "OptiTrack "/1(OptiTrack) -> optiTrack/1, OptiTrack/1

== system IARC_Nonlinear_Sensors/Signal generator/X_des ==
  Add : Sum  Inputs=+++++
  Rate Transition1 : RateTransition  Commented=on
  Repeating Sequence Stair1 : simulink/Sources/Repeating Sequence Stair  Commented=on  OutValues=[0 0 1 0 0 -1 0 1].'  tsamp=T*500*5  OutMin=[]  OutMax=[]  OutDataTypeStr=double  OutputDataTypeScalingMode=double  OutDataType=fixdt(0,8)  ConRadixGroup=Best Precision: Vector-wise  OutScaling=2^-12
  x_des1 : Step  Time=15  After=1*0  SampleTime=0
  x_des2 : Step  Time=10  After=1*2  SampleTime=0
  "x_des2 " : Step  Time=40  After=-1*2  SampleTime=0
  x_des2 1 : Step  Time=45  After=-1*0  SampleTime=0
  x_des : Outport
  wires:
  Repeating Sequence Stair1/1 -> Rate Transition1/1  "y_des"
  x_des1/1 -> Add/2  "x_des"
  Add/1 -> x_des/1  "x_des"
  "x_des2 "/1 -> Add/3
  x_des2/1 -> Add/1
  x_des2 1/1 -> Add/4

== system IARC_Nonlinear_Sensors/Signal generator/Y_des ==
  Add : Sum  Inputs=+++++
  Rate Transition1 : RateTransition
  Repeating Sequence Stair1 : simulink/Sources/Repeating Sequence Stair  OutValues=[0 0 1 0 0 -1 0 1].'  tsamp=T*500*5  OutMin=[]  OutMax=[]  OutDataTypeStr=double  OutputDataTypeScalingMode=double  OutDataType=fixdt(0,8)  ConRadixGroup=Best Precision: Vector-wise  OutScaling=2^-12
  y_des1 : Step  Time=15  SampleTime=0
  y_des2 : Step  Time=10  After=1*0  SampleTime=0
  "y_des2 " : Step  Time=40  After=-1*0  SampleTime=0
  y_des2 1 : Step  Time=45  After=-1  SampleTime=0
  x_des : Outport
  wires:
  y_des2 1/1 -> Add/4
  y_des2/1 -> Add/1
  "y_des2 "/1 -> Add/3
  Add/1 -> x_des/1  "x_des"
  y_des1/1 -> Add/2  "x_des"
  Repeating Sequence Stair1/1 -> Rate Transition1/1  "y_des"

== system IARC_Nonlinear_Sensors/Signal generator/Yaw_des ==
  Repeating Sequence Interpolated6 : simulink/Sources/Repeating Sequence Interpolated  OutValues=90*pi/180*[0 0 1 1 0 0 -0.5 -0.5 0 0].'  TimeValues=[0 10 10.1 15 15.1 20 20.1 25 25.1 30].'  LookUpMeth=Interpolation-Use End Values  tsamp=T  OutMin=[]  OutMax=[]  OutDataTypeStr=double  OutputDataTypeScalingMode=double  OutDataType=fixdt(0,8)  OutScaling=2^-10
  Sum3 : Sum  Inputs=++|
  Sum4 : Sum  Inputs=++|
  psi_des : Step  Time=55  After=-10*pi/180  SampleTime=0
  psi_des1 : Step  Time=50  After=10*pi/180  SampleTime=0
  psi_des2 : Step  Time=0  After=0*pi/180  SampleTime=0
  Out1 : Outport
  wires:
  psi_des1/1 -> Sum3/1
  psi_des/1 -> Sum3/2  "yaw_des"
  Sum3/1 -> Sum4/1  "yaw_des"
  Repeating Sequence Interpolated6/1 -> ?  "yaw_des"
  psi_des2/1 -> Out1/1

== system IARC_Nonlinear_Sensors/Signal generator/Z_des ==
  Position3 : Scope  Commented=on
  Sine Wave : Sin  Amplitude=0  Frequency=2*pi  SampleTime=0
  Sum : Sum  Inputs=++|
  Sum1 : Sum  Inputs=+++|+
  z_des1 : Step  Time=5  SampleTime=0
  "z_des2 " : Step  Commented=on  Time=10  After=0.8  SampleTime=0
  z_des3 : Step  Time=20  After=-1  SampleTime=0
  z_des4 : Step  Time=30  SampleTime=0
  z_des : Outport
  wires:
  Sine Wave/1 -> Sum/1
  "z_des2 "/1 -> ?
  Sum1/1 -> Position3/1, Sum/2  "z_des"
  Sum/1 -> z_des/1  "z_des"
  z_des1/1 -> Sum1/1
  z_des3/1 -> Sum1/3
  z_des4/1 -> Sum1/4

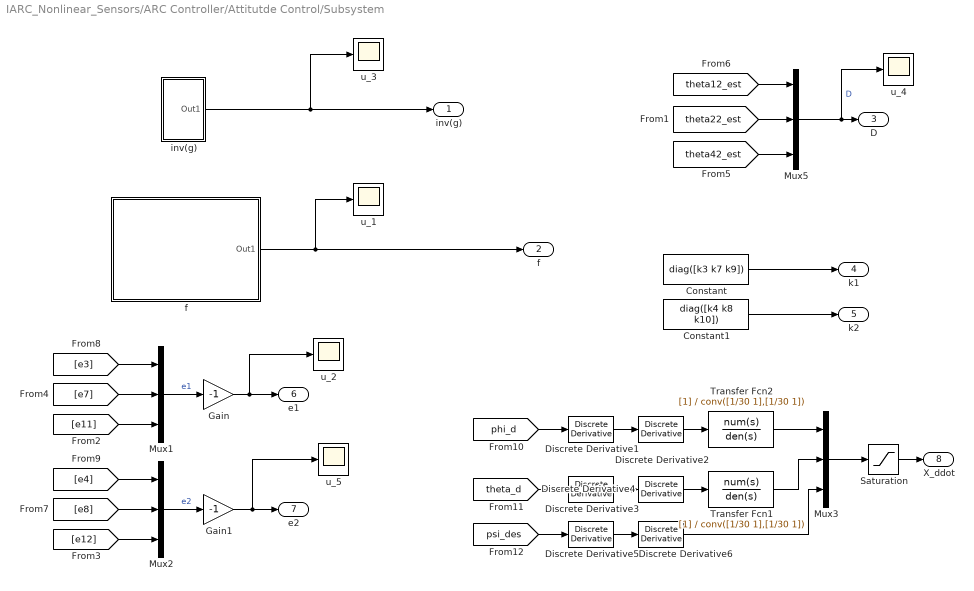
== system IARC_Nonlinear_Sensors/ARC Controller/Attitutde Control/Subsystem ==
  Constant : Constant  Value=diag([k3 k7 k9])
  Constant1 : Constant  Value=diag([k4 k8 k10])
  Discrete Derivative{1..6} (6 alike) : simulink/Discrete/Discrete Derivative  gainval=1.0  ICPrevScaledInput=0.0  OutMin=[]  OutMax=[]  OutDataType=fixdt(1, 16)  OutScaling=2^-10  DoSatur=off
  Gain : Gain  Gain=-1
  Gain1 : Gain  Gain=-1
  Mux{1..3,5} (4 alike) : Mux  Inputs=3
  Saturation : Saturate  UpperLimit=[10]  LowerLimit=[-10]
  Transfer Fcn1 : TransferFcn  Denominator=conv([1/30 1],[1/30 1])
  Transfer Fcn2 : TransferFcn  Denominator=conv([1/30 1],[1/30 1])
  f : Subsystem
  inv(g) : Subsystem
  u_{1..5} (5 alike) : Scope
  "inv(g) " : Outport
  "f " : Outport  Port=2
  D : Outport  Port=3
  k1 : Outport  Port=4
  k2 : Outport  Port=5
  e1 : Outport  Port=6
  e2 : Outport  Port=7
  X_ddot : Outport  Port=8
  wires:
  [theta42_est] -> Mux5/3
  [theta22_est] -> Mux5/2
  [theta12_est] -> Mux5/1
  Mux5/1 -> u_4/1, D/1  "D"
  f/1(Out1) -> u_1/1, "f "/1
  inv(g)/1(Out1) -> u_3/1, "inv(g) "/1
  [e3] -> Mux1/1
  [e7] -> Mux1/2
  [e11] -> Mux1/3
  [e4] -> Mux2/1
  [e8] -> Mux2/2
  [e12] -> Mux2/3
  Mux1/1 -> Gain/1  "e1"
  Mux2/1 -> Gain1/1  "e2"
  Constant/1 -> k1/1
  Constant1/1 -> k2/1
  Gain/1 -> u_2/1, e1/1
  Gain1/1 -> u_5/1, e2/1
  Discrete Derivative1/1 -> Discrete Derivative2/1
  Discrete Derivative3/1 -> Discrete Derivative4/1
  Mux3/1 -> Saturation/1
  Discrete Derivative5/1 -> Discrete Derivative6/1
  [psi_des] -> Discrete Derivative5/1
  Discrete Derivative6/1 -> Mux3/3
  Saturation/1 -> X_ddot/1
  [phi_d] -> Discrete Derivative1/1
  [theta_d] -> Discrete Derivative3/1
  Discrete Derivative4/1 -> Transfer Fcn1/1
  Discrete Derivative2/1 -> Transfer Fcn2/1
  Transfer Fcn2/1 -> Mux3/1
  Transfer Fcn1/1 -> Mux3/2

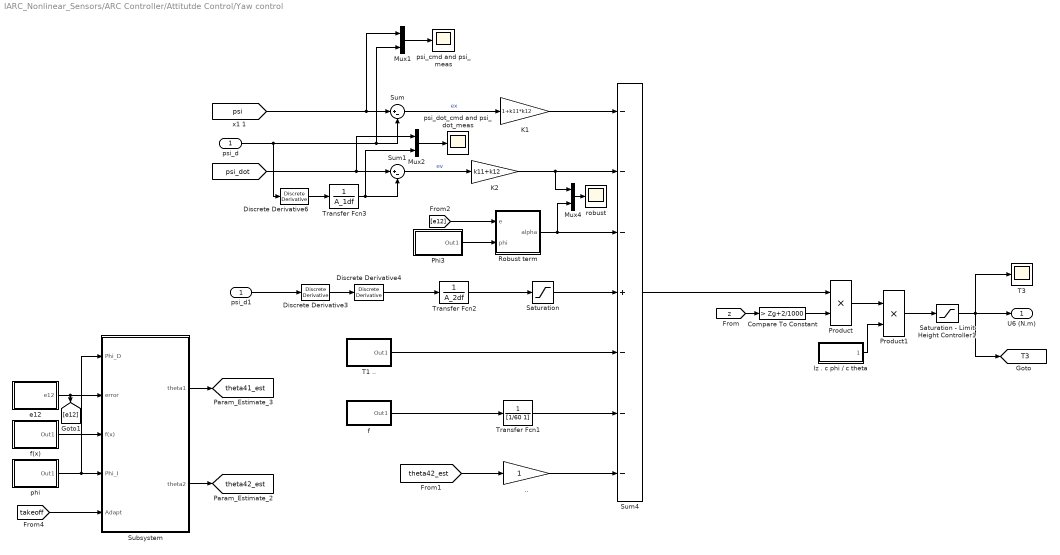
== system IARC_Nonlinear_Sensors/ARC Controller/Attitutde Control/Yaw control ==
  psi_d : Inport
  .. : Gain
  Compare To Constant : simulink/Logic and Bit Operations/Compare To Constant  relop=>  const=Zg+2/1000  OutDataTypeStr=uint8  ZeroCross=off
  Discrete Derivative3 : simulink/Discrete/Discrete Derivative  gainval=1.0  ICPrevScaledInput=0.0  OutMin=[]  OutMax=[]  OutDataType=fixdt(1, 16)  OutScaling=2^-10  DoSatur=off
  Discrete Derivative4 : simulink/Discrete/Discrete Derivative  gainval=1.0  ICPrevScaledInput=0.0  OutMin=[]  OutMax=[]  OutDataType=fixdt(1, 16)  OutScaling=2^-10  DoSatur=off
  Discrete Derivative6 : simulink/Discrete/Discrete Derivative  gainval=1.0  ICPrevScaledInput=0.0  OutMin=[]  OutMax=[]  OutDataType=fixdt(1, 16)  OutScaling=2^-10  DoSatur=off
  Iz . c phi / c theta : Subsystem
  K1 : Gain  Gain=1+k11*k12
  K2 : Gain  Gain=k11+k12
  Mux1 : Mux  Inputs=2
  Mux2 : Mux  Inputs=2
  Mux4 : Mux  Inputs=2
  Phi3 : Subsystem
  Product : Product  Inputs=**
  Product1 : Product
  Robust term : Subsystem  mask(Robust_Block){theta_max=theta3_Max, theta_min=theta3_Min, epsilon=Epsilon3, delta=delta3}
      mask prompts: theta_max "Maximum parameters vector value:"; theta_min "Minimum parameters vector value:"; epsilon "Error bound Coefficient:"; delta "Uncertain Nonlinearities Bound:"
      mask help: Computes the nonlinear robust feedback.
      mask Help:
      | h^2=(theta_max-theta_min)^2*phi^2+delta^2
      | u = h/(4epsilon) )e/theta
      mask Display:
      | port_label('input',1,'e','texmode','on')
      | port_label('input',2,'\phi','texmode','on')
      | 
      | port_label('output',1,'u_{s2}','texmode','on')
  Saturation : Saturate  UpperLimit=[10]  LowerLimit=[-10]
  Saturation - Limit Height Controller1 : Saturate  UpperLimit=0.8  LowerLimit=-0.8
  Subsystem : Subsystem
  Sum : Sum  Inputs=|+-
  Sum1 : Sum  Inputs=|+-
  Sum4 : Sum  Inputs=---+---
  T1 .. : Subsystem
  "T3 " : Scope
  Transfer Fcn1 : TransferFcn  Denominator=[1/60 1]
  Transfer Fcn2 : TransferFcn  Denominator=A_2df
  Transfer Fcn3 : TransferFcn  Denominator=A_1df
  e12 : Subsystem
  f : Subsystem
  f(x) : Subsystem
  phi : Subsystem
  psi_cmd and psi_meas : Scope
  psi_d1 : InportShadow
  psi_dot_cmd and psi_dot_meas : Scope
  robust : Scope
  U6 (N.m) : Outport
  tag scope: T3=global, theta41_est=global, theta42_est=global
  wires:
  Transfer Fcn2/1 -> Saturation/1
  Mux1/1 -> psi_cmd and psi_meas/1
  Sum/1 -> K1/1  "ex"
  [psi] -> Mux1/1, Sum/1
  [z] -> Compare To Constant/1
  Compare To Constant/1 -> Product/2
  Sum4/1 -> Product/1
  psi_d1/1 -> Discrete Derivative3/1
  Discrete Derivative3/1 -> Discrete Derivative4/1
  K1/1 -> Sum4/1
  K2/1 -> Mux4/1, Sum4/2
  Discrete Derivative4/1 -> Transfer Fcn2/1
  phi/1(Out1) -> Subsystem/1(Phi_D), Subsystem/4(Phi_I)
  f(x)/1(Out1) -> Subsystem/3(f(x))
  Discrete Derivative6/1 -> Transfer Fcn3/1
  [psi_dot] -> Mux2/1, Sum1/1
  Mux2/1 -> psi_dot_cmd and psi_dot_meas/1
  e12/1(e12) -> Subsystem/2(error), [e12]
  Iz . c phi / c theta/1(" ") -> Product1/2
  ../1 -> Sum4/7
  Product/1 -> Product1/1
  Phi3/1(Out1) -> Robust term/2(phi)
  Sum1/1 -> K2/1  "ev"
  [e12] -> Robust term/1(e)
  Robust term/1(alpha) -> Mux4/2, Sum4/3
  Product1/1 -> Saturation - Limit Height Controller1/1
  psi_d/1 -> Discrete Derivative6/1, Mux1/2, Sum/2
  [theta42_est] -> ../1
  T1 ../1(Out1) -> Sum4/5
  f/1(Out1) -> Transfer Fcn1/1
  Transfer Fcn3/1 -> Sum1/2, Mux2/2
  Saturation/1 -> Sum4/4
  Subsystem/1(theta1) -> [theta41_est]
  Subsystem/2(theta2) -> [theta42_est]
  [takeoff] -> Subsystem/5(Adapt)
  Saturation - Limit Height Controller1/1 -> "T3 "/1, [T3], U6 (N.m)/1
  Transfer Fcn1/1 -> Sum4/6
  Mux4/1 -> robust/1

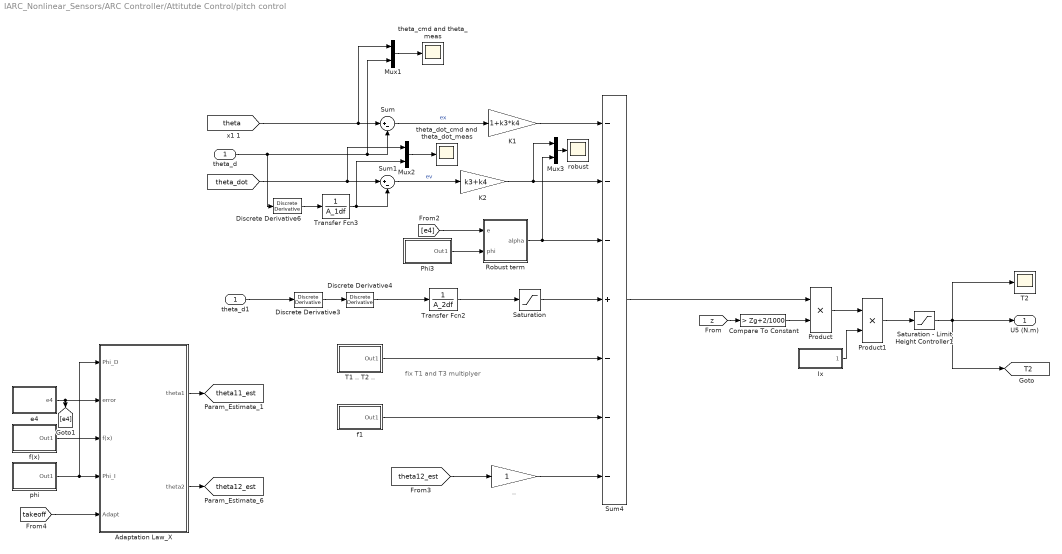
== system IARC_Nonlinear_Sensors/ARC Controller/Attitutde Control/pitch control ==
  note: fix T1 and T3 multiplyer
  theta_d : Inport
  .. : Gain
  Adaptation Law_X : Subsystem
  Compare To Constant : simulink/Logic and Bit Operations/Compare To Constant  relop=>  const=Zg+2/1000  OutDataTypeStr=uint8  ZeroCross=off
  Discrete Derivative3 : simulink/Discrete/Discrete Derivative  gainval=1.0  ICPrevScaledInput=0.0  OutMin=[]  OutMax=[]  OutDataType=fixdt(1, 16)  OutScaling=2^-10  DoSatur=off
  Discrete Derivative4 : simulink/Discrete/Discrete Derivative  gainval=1.0  ICPrevScaledInput=0.0  OutMin=[]  OutMax=[]  OutDataType=fixdt(1, 16)  OutScaling=2^-10  DoSatur=off
  Discrete Derivative6 : simulink/Discrete/Discrete Derivative  gainval=1.0  ICPrevScaledInput=0.0  OutMin=[]  OutMax=[]  OutDataType=fixdt(1, 16)  OutScaling=2^-10  DoSatur=off
  Ix : Subsystem
  K1 : Gain  Gain=1+k3*k4
  K2 : Gain  Gain=k3+k4
  Mux1 : Mux  Inputs=2
  Mux2 : Mux  Inputs=2
  Mux3 : Mux  Inputs=2
  Phi3 : Subsystem
  Product : Product  Inputs=**
  Product1 : Product
  Robust term : Subsystem  mask(Robust_Block){theta_max=theta3_Max, theta_min=theta3_Min, epsilon=Epsilon3, delta=delta3}
      mask prompts: theta_max "Maximum parameters vector value:"; theta_min "Minimum parameters vector value:"; epsilon "Error bound Coefficient:"; delta "Uncertain Nonlinearities Bound:"
      mask help: Computes the nonlinear robust feedback.
      mask Help:
      | h^2=(theta_max-theta_min)^2*phi^2+delta^2
      | u = h/(4epsilon) )e/theta
      mask Display:
      | port_label('input',1,'e','texmode','on')
      | port_label('input',2,'\phi','texmode','on')
      | 
      | port_label('output',1,'u_{s2}','texmode','on')
  Saturation : Saturate  UpperLimit=[10]  LowerLimit=[-10]
  Saturation - Limit Height Controller1 : Saturate  UpperLimit=0.8  LowerLimit=-0.8
  Sum : Sum  Inputs=|+-
  Sum1 : Sum  Inputs=|+-
  Sum4 : Sum  Inputs=---+---
  T1 .. T2 .. : Subsystem
  "T2 " : Scope
  Transfer Fcn2 : TransferFcn  Denominator=A_2df
  Transfer Fcn3 : TransferFcn  Denominator=A_1df
  e4 : Subsystem
  f(x) : Subsystem
  f1 : Subsystem
  phi : Subsystem
  robust : Scope
  theta_cmd and theta_meas : Scope
  theta_d1 : InportShadow
  theta_dot_cmd and theta_dot_meas : Scope
  U5 (N.m) : Outport
  tag scope: T2=global, theta11_est=global, theta12_est=global
  wires:
  Saturation/1 -> Sum4/4
  Transfer Fcn3/1 -> Mux2/2, Sum1/2
  f1/1(Out1) -> Sum4/6
  T1 .. T2 ../1(Out1) -> Sum4/5
  [theta12_est] -> ../1
  theta_d/1 -> Sum/2, Mux1/2, Discrete Derivative6/1
  Product1/1 -> Saturation - Limit Height Controller1/1
  Saturation - Limit Height Controller1/1 -> "T2 "/1, [T2], U5 (N.m)/1
  Robust term/1(alpha) -> Mux3/2, Sum4/3
  [e4] -> Robust term/1(e)
  Sum1/1 -> K2/1  "ev"
  Phi3/1(Out1) -> Robust term/2(phi)
  Product/1 -> Product1/1
  ../1 -> Sum4/7
  Adaptation Law_X/1(theta1) -> [theta11_est]
  Ix/1(" ") -> Product1/2
  Adaptation Law_X/2(theta2) -> [theta12_est]
  e4/1(e4) -> Adaptation Law_X/2(error), [e4]
  Mux2/1 -> theta_dot_cmd and theta_dot_meas/1
  [theta_dot] -> Sum1/1, Mux2/1
  Discrete Derivative6/1 -> Transfer Fcn3/1
  [takeoff] -> Adaptation Law_X/5(Adapt)
  phi/1(Out1) -> Adaptation Law_X/4(Phi_I), Adaptation Law_X/1(Phi_D)
  Discrete Derivative4/1 -> Transfer Fcn2/1
  K2/1 -> Mux3/1, Sum4/2
  K1/1 -> Sum4/1
  Discrete Derivative3/1 -> Discrete Derivative4/1
  theta_d1/1 -> Discrete Derivative3/1
  Sum4/1 -> Product/1
  Compare To Constant/1 -> Product/2
  [z] -> Compare To Constant/1
  [theta] -> Sum/1, Mux1/1
  Sum/1 -> K1/1  "ex"
  Mux1/1 -> theta_cmd and theta_meas/1
  Transfer Fcn2/1 -> Saturation/1
  f(x)/1(Out1) -> Adaptation Law_X/3(f(x))
  Mux3/1 -> robust/1
